simulink model "crc8_locator"  (R2024b)
settings: Solver=FixedStepDiscrete  StartTime=0.0  StopTime=10  FixedStep=1  RelTol=1e-3
settings Model: Creator=samue  LastModifiedBy=samue
settings OptimizationCC: BlockReduction=off  ConditionallyExecuteInputs=off  DefaultParameterBehavior=Inlined
settings DebuggingCC: AlgebraicLoopMsg=error
settings HardwareCC: ProdBitPerPointer=32  ProdBitPerSizeT=32  ProdBitPerPtrDiffT=32  ProdLargestAtomicFloat=None  ProdIntDivRoundTo=Undefined  ProdEndianess=Unspecified  ProdWordSize=32  ProdHWDeviceType=ASIC/FPGA->ASIC/FPGA  TargetBitPerPointer=64  TargetBitPerSizeT=64  TargetBitPerPtrDiffT=64  TargetLongLongMode=on  TargetIntDivRoundTo=Zero  TargetEndianess=LittleEndian  TargetWordSize=64  TargetHWDeviceType=Custom Processor->MATLAB Host Computer  ProdEqTarget=off

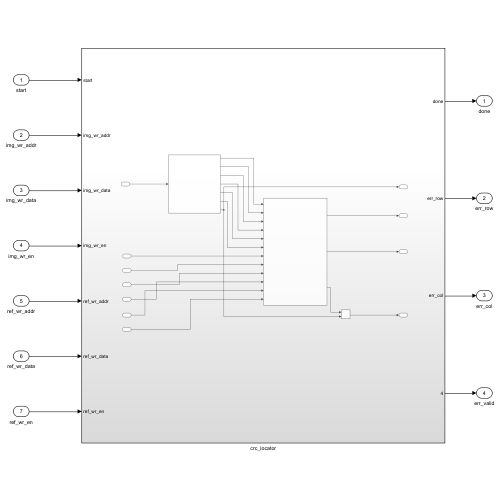
[thumbnail: Simulink's stored preview of the top-level diagram]
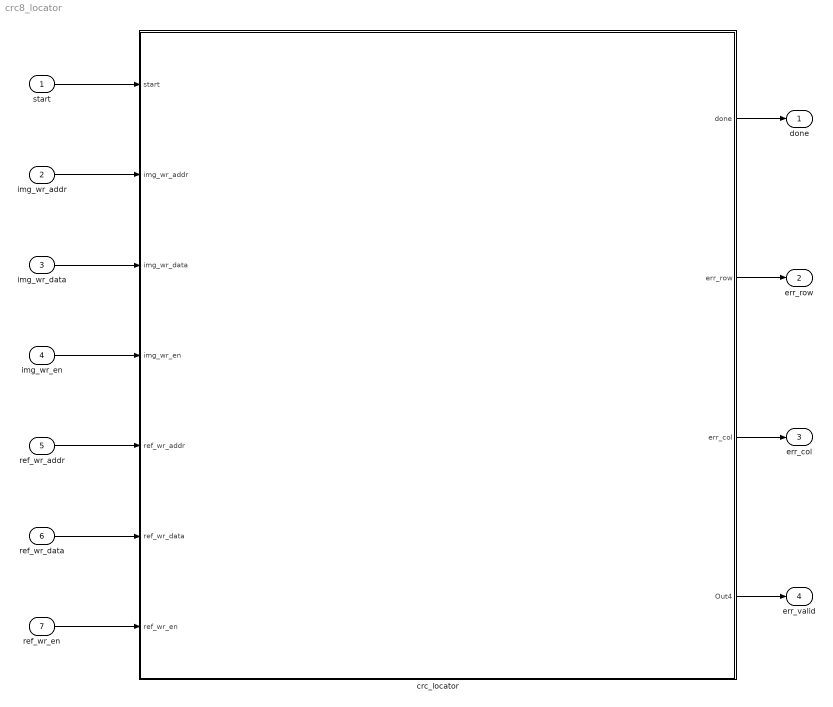
== system crc8_locator ==
  start : Inport  OutDataTypeStr=boolean  PortDimensions=1
  img_wr_addr : Inport  Port=2  OutDataTypeStr=uint16  PortDimensions=1
  img_wr_data : Inport  Port=3  OutDataTypeStr=uint8  PortDimensions=1
  img_wr_en : Inport  Port=4  OutDataTypeStr=boolean  PortDimensions=1
  ref_wr_addr : Inport  Port=5  OutDataTypeStr=uint16  PortDimensions=1
  ref_wr_data : Inport  Port=6  OutDataTypeStr=uint8  PortDimensions=1
  ref_wr_en : Inport  Port=7  OutDataTypeStr=boolean  PortDimensions=1
  crc_locator : Subsystem
  done : Outport
  err_row : Outport  Port=2
  err_col : Outport  Port=3
  err_valid : Outport  Port=4
  wires:
  start/1 -> crc_locator/1(start)
  img_wr_addr/1 -> crc_locator/2(img_wr_addr)
  img_wr_data/1 -> crc_locator/3(img_wr_data)
  crc_locator/1(done) -> done/1
  crc_locator/4(Out4) -> err_valid/1
  img_wr_en/1 -> crc_locator/4(img_wr_en)
  ref_wr_addr/1 -> crc_locator/5(ref_wr_addr)
  ref_wr_data/1 -> crc_locator/6(ref_wr_data)
  ref_wr_en/1 -> crc_locator/7(ref_wr_en)
  crc_locator/2(err_row) -> err_row/1
  crc_locator/3(err_col) -> err_col/1

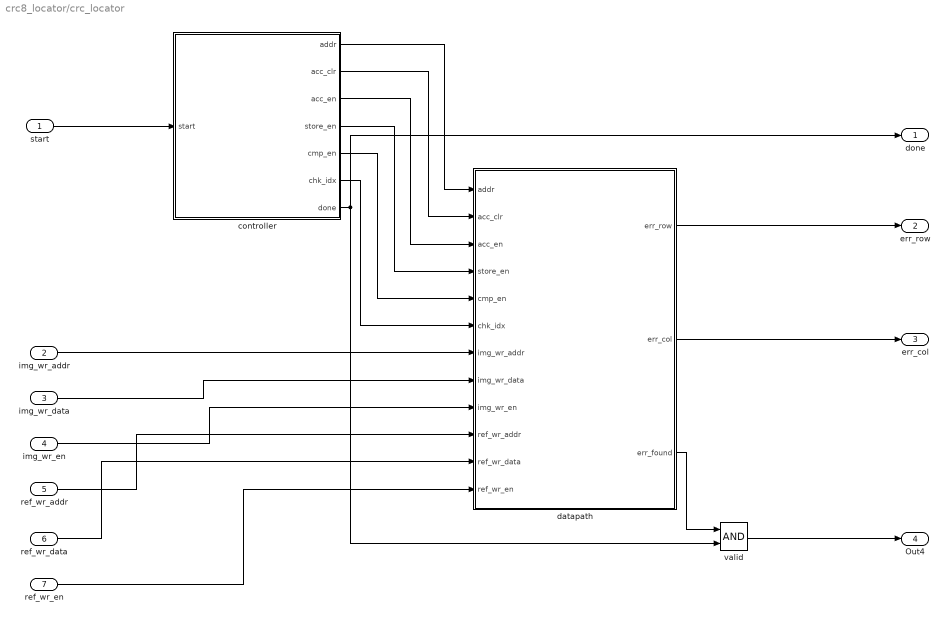
== system crc8_locator/crc_locator ==
  start : Inport
  img_wr_addr : Inport  Port=2
  img_wr_data : Inport  Port=3
  img_wr_en : Inport  Port=4
  ref_wr_addr : Inport  Port=5
  ref_wr_data : Inport  Port=6
  ref_wr_en : Inport  Port=7
  controller : MATLAB Function  TreatAsAtomicUnit=on
  datapath : Subsystem
  valid : Logic  AllPortsSameDT=off  OutDataTypeStr=boolean
  done : Outport
  err_row : Outport  Port=2
  err_col : Outport  Port=3
  Out4 : Outport  Port=4
  wires:
  img_wr_data/1 -> datapath/8(img_wr_data)
  controller/5(cmp_en) -> datapath/5(cmp_en)
  controller/1(addr) -> datapath/1(addr)
  start/1 -> controller/1(start)
  controller/2(acc_clr) -> datapath/2(acc_clr)
  ref_wr_en/1 -> datapath/12(ref_wr_en)
  controller/6(chk_idx) -> datapath/6(chk_idx)
  controller/4(store_en) -> datapath/4(store_en)
  controller/3(acc_en) -> datapath/3(acc_en)
  datapath/3(err_found) -> valid/1
  img_wr_addr/1 -> datapath/7(img_wr_addr)
  controller/7(done) -> done/1, valid/2
  ref_wr_data/1 -> datapath/11(ref_wr_data)
  datapath/1(err_row) -> err_row/1
  datapath/2(err_col) -> err_col/1
  ref_wr_addr/1 -> datapath/10(ref_wr_addr)
  img_wr_en/1 -> datapath/9(img_wr_en)
  valid/1 -> Out4/1

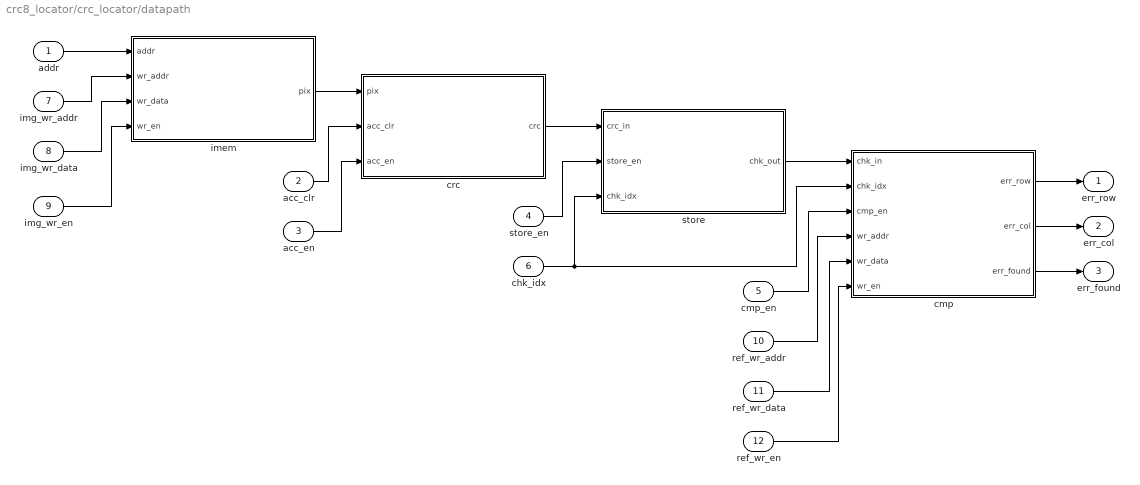
== system crc8_locator/crc_locator/datapath ==
  addr : Inport  OutDataTypeStr=uint16  PortDimensions=1
  acc_clr : Inport  Port=2  OutDataTypeStr=boolean  PortDimensions=1
  acc_en : Inport  Port=3  OutDataTypeStr=boolean  PortDimensions=1
  store_en : Inport  Port=4  OutDataTypeStr=boolean  PortDimensions=1
  cmp_en : Inport  Port=5  OutDataTypeStr=boolean  PortDimensions=1
  chk_idx : Inport  Port=6  OutDataTypeStr=uint8  PortDimensions=1
  img_wr_addr : Inport  Port=7  OutDataTypeStr=uint16  PortDimensions=1
  img_wr_data : Inport  Port=8  OutDataTypeStr=uint8  PortDimensions=1
  img_wr_en : Inport  Port=9  OutDataTypeStr=boolean  PortDimensions=1
  ref_wr_addr : Inport  Port=10  OutDataTypeStr=uint16  PortDimensions=1
  ref_wr_data : Inport  Port=11  OutDataTypeStr=uint8  PortDimensions=1
  ref_wr_en : Inport  Port=12  OutDataTypeStr=boolean  PortDimensions=1
  cmp : MATLAB Function  TreatAsAtomicUnit=on
  crc : MATLAB Function  TreatAsAtomicUnit=on
  imem : MATLAB Function  TreatAsAtomicUnit=on
  store : MATLAB Function  TreatAsAtomicUnit=on
  err_row : Outport
  err_col : Outport  Port=2
  err_found : Outport  Port=3
  wires:
  acc_clr/1 -> crc/2(acc_clr)
  addr/1 -> imem/1(addr)
  img_wr_addr/1 -> imem/2(wr_addr)
  imem/1(pix) -> crc/1(pix)
  img_wr_en/1 -> imem/4(wr_en)
  ref_wr_addr/1 -> cmp/4(wr_addr)
  img_wr_data/1 -> imem/3(wr_data)
  cmp_en/1 -> cmp/3(cmp_en)
  acc_en/1 -> crc/3(acc_en)
  crc/1(crc) -> store/1(crc_in)
  store_en/1 -> store/2(store_en)
  chk_idx/1 -> cmp/2(chk_idx), store/3(chk_idx)
  store/1(chk_out) -> cmp/1(chk_in)
  ref_wr_data/1 -> cmp/5(wr_data)
  ref_wr_en/1 -> cmp/6(wr_en)
  cmp/1(err_row) -> err_row/1
  cmp/2(err_col) -> err_col/1
  cmp/3(err_found) -> err_found/1

== matlab function crc8_locator/crc_locator/datapath/crc ==
  data: pix input; crc output; acc_clr input; acc_en input
function crc = dp_crc(pix, acc_clr, acc_en)
% CRC8 accumulator

%#codegen

    persistent creg
    if isempty(creg)
        creg = uint8(0);
    end

    crc = creg;

    if acc_clr
        creg = uint8(0);
    elseif acc_en
        c = bitxor(creg, pix);
        for n = 1:8
            if bitand(c, uint8(128)) ~= 0
                c = bitxor(bitshift(c, 1), uint8(7));
            else
                c = bitshift(c, 1);
            end
        end
        creg = c;
    end
end

== matlab function crc8_locator/crc_locator/datapath/imem ==
  data: addr input; pix output; wr_addr input; wr_data input; wr_en input
function pix = dp_imem(addr, wr_addr, wr_data, wr_en)
% Image memory: 1024 x 8 with a two-cycle read

%#codegen

    persistent mem stage1 pixq
    if isempty(mem)
        mem    = zeros(1024, 1, 'uint8');
        stage1 = uint8(0);
        pixq   = uint8(0);
    end

    pix = pixq;                         % the registers as they stand on entry

    pixq   = stage1;                    % updated on this clock edge
    stage1 = mem(addr + uint16(1));
    if wr_en
        mem(wr_addr + uint16(1)) = wr_data;
    end
end

== matlab function crc8_locator/crc_locator/datapath/store ==
  data: crc_in input; chk_out output; store_en input; chk_idx input
function chk_out = dp_store(crc_in, store_en, chk_idx)
% Check store: 64 x 8, written at STORE, read at CMP

%#codegen

    persistent chk
    if isempty(chk)
        chk = zeros(64, 1, 'uint8');
    end

    chk_out = chk(chk_idx + uint8(1));

    if store_en
        chk(chk_idx + uint8(1)) = crc_in;
    end
end

== matlab function crc8_locator/crc_locator/datapath/cmp ==
  data: chk_in input; err_row output; chk_idx input; cmp_en input; wr_addr input; wr_data input; wr_en input; err_col output; err_found output
function [err_row, err_col, err_found] = dp_cmp(chk_in, chk_idx, cmp_en, ...
                                                wr_addr, wr_data, wr_en)
% Comparator and error registers

%#codegen

    persistent ref er ec rf cf
    if isempty(ref)
        ref = zeros(64, 1, 'uint8');
        er  = uint8(0);
        ec  = uint8(0);
        rf  = false;
        cf  = false;
    end

    err_row   = er;
    err_col   = ec;
    err_found = rf && cf;

    if cmp_en
        % clear registers at very start of a run, before checks happen
        if chk_idx == uint8(0)
            er = uint8(0);
            ec = uint8(0);
            rf = false;
            cf = false;
        end

        is_col = bitand(chk_idx, uint8(32)) ~= 0;
        line   = bitand(chk_idx, uint8(31));
        if chk_in ~= ref(chk_idx + uint8(1))
            if is_col
                if ~cf
                    ec = line;
                    cf = true;
                end
            else
                if ~rf
                    er = line;
                    rf = true;
                end
            end
        end
    end

    if wr_en
        ref(wr_addr + uint16(1)) = wr_data;
    end
end

== matlab function crc8_locator/crc_locator/controller ==
  data: start input; addr output; acc_clr output; acc_en output; store_en output; cmp_en output; chk_idx output; done output
function [addr, acc_clr, acc_en, store_en, cmp_en, chk_idx, done] ...
         = crc_ctrl(start)
% Controller for the row/column CRC error locator

%#codegen

    persistent state i k pass
    if isempty(state)
        state = ctrl_state.IDLE;
        i     = uint8(0);      % element within the current line, 0-31
        k     = uint8(0);      % line index, 0-31; also compare index, 0-63
        pass  = false;         % false = rows, true = columns
    end

    % default outputs
    addr     = uint16(0);
    acc_clr  = false;
    acc_en   = false;
    store_en = false;
    cmp_en   = false;
    chk_idx  = uint8(0);
    done     = false;

    switch state

        case ctrl_state.IDLE
            i    = uint8(0);
            k    = uint8(0);
            pass = false;
            if start
                state = ctrl_state.LOAD;
            end

        case ctrl_state.LOAD
            addr    = elem_addr(i, k, pass);
            acc_clr = (i == uint8(0));
            state   = ctrl_state.HOLD;

        case ctrl_state.HOLD
            addr  = elem_addr(i, k, pass);
            state = ctrl_state.ACC;

        case ctrl_state.ACC
            acc_en = true;
            if i == uint8(31)
                i     = uint8(0);
                state = ctrl_state.STORE;
            else
                i     = i + uint8(1);
                state = ctrl_state.LOAD;
            end

        case ctrl_state.STORE
            store_en = true;
            chk_idx  = check_index(k, pass);
            if k == uint8(31)
                k     = uint8(0);
                state = ctrl_state.SWAP;
            else
                k     = k + uint8(1);
                state = ctrl_state.LOAD;
            end

        case ctrl_state.SWAP
            k = uint8(0);
            if pass
                state = ctrl_state.CMP;
            else
                pass  = true;
                state = ctrl_state.LOAD;
            end

        case ctrl_state.CMP
            cmp_en  = true;
            chk_idx = k;
            if k == uint8(63)
                state = ctrl_state.DONE;
            else
                k = k + uint8(1);
            end

        case ctrl_state.DONE
            done = true;
            if ~start
                state = ctrl_state.IDLE;
            end

        otherwise
            state = ctrl_state.IDLE;
    end
end

% -------------------------------------------------------------------------
function a = elem_addr(i, k, pass)
    if pass
        a = uint16(i) * uint16(32) + uint16(k);   % column k, going down
    else
        a = uint16(k) * uint16(32) + uint16(i);   % row k, going across
    end
end

% -------------------------------------------------------------------------
function x = check_index(k, pass)
    if pass
        x = k + uint8(32);
    else
        x = k;
    end
end
